simulink model "Dpt_S_Fun_1_C"  (Simulink 4.00)
settings: Solver=ode45  SolverMode=SingleTasking  StartTime=0.0  StopTime=0.4  FixedStep=0.01  MaxStep=0.001  RelTol=1e-3  AbsTol=1e-3
PreLoadFcn:
  | Load_Param_1
undefined symbols (not defined in the file): Cm, Cw, Fi, J, L, Mnabr, R, Tnabr, V
settings Model: SaveTime=off  SaveOutput=off  LimitDataPoints=off  RTWTemplateMakefile=grt_vc.tmf  BlockReductionOpt=off

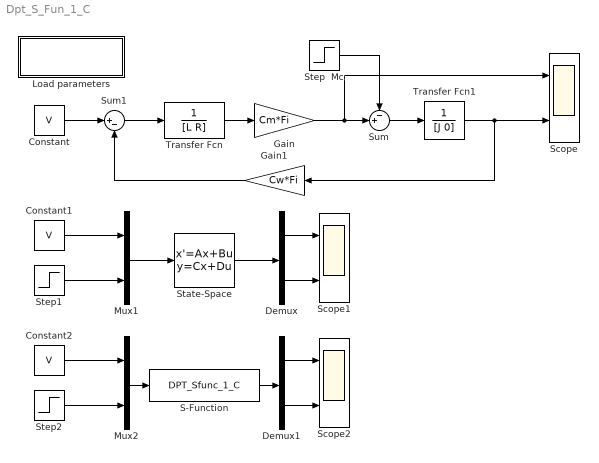
== system Dpt_S_Fun_1_C ==
  Constant : Constant  Value=V
  Constant1 : Constant  Value=V
  Constant2 : Constant  Value=V
  Demux : Demux  Outputs=2  BusSelectionMode=off
  Demux1 : Demux  Outputs=2  BusSelectionMode=off
  Gain : Gain  Gain=Cm*Fi  Multiplication=Element-wise(K.*u)  SaturateOnIntegerOverflow=on
  Gain1 : Gain  Orientation=left  Gain=Cw*Fi  Multiplication=Element-wise(K.*u)  SaturateOnIntegerOverflow=on
  Load parameters : Subsystem
      settings: OpenFcn=Load_Param_1  RTWFcnNameOpts=Auto  RTWFileNameOpts=Auto
      mask Help: Click here to save t and yout in an ascii data file called temp.dat
      mask Display: disp('Click here to\n load parameters')
  Mux1 : Mux  Inputs=2
  Mux2 : Mux  Inputs=2
  S-Function : S-Function  FunctionName=DPT_Sfunc_1_C  Parameters=L,R,J,Cm,Cw,Fi  PortCounts=[]  SFunctionModules=''
  Scope : Scope  NumInputPorts=2
      settings: TimeRange=0.4  YMin=-3286.73~0  YMax=12937.8~30  SaveToWorkspace=off  SaveName=ScopeData  LimitDataPoints=on  MaxDataPoints=5000
  Scope1 : Scope  NumInputPorts=2
      settings: TimeRange=0.4  YMin=-3286.73~0  YMax=12937.8~30  SaveToWorkspace=off  LimitDataPoints=on  MaxDataPoints=5000
  Scope2 : Scope  NumInputPorts=2
      settings: TimeRange=0.4  YMin=-3286.73~0  YMax=12937.8~30  SaveToWorkspace=off  SaveName=ScopeData2  LimitDataPoints=on  MaxDataPoints=5000
  State-Space : StateSpace  A=[-R/L -Cw*Fi/L;Cm*Fi/J 0]  B=[1/L 0;0 -1/J]  C=[Cm*Fi 0;0 1]  D=[0 0;0 0]  X0=[0;0]  AbsoluteTolerance=auto  Realization=auto
  Step  Mc : Step  Time=Tnabr  Before=0  After=Mnabr  SampleTime=0
  Step1 : Step  Time=Tnabr  Before=0  After=Mnabr  SampleTime=0
  Step2 : Step  Time=Tnabr  Before=0  After=Mnabr  SampleTime=0
  Sum : Sum  Inputs=-+|  SaturateOnIntegerOverflow=on
  Sum1 : Sum  Inputs=|+-  SaturateOnIntegerOverflow=on
  Transfer Fcn : TransferFcn  Numerator=[1]  Denominator=[L R]  AbsoluteTolerance=auto  Realization=auto
  Transfer Fcn1 : TransferFcn  Numerator=[1]  Denominator=[J 0]  AbsoluteTolerance=auto  Realization=auto
  wires:
  Constant2/1 -> Mux2/1
  Step2/1 -> Mux2/2
  Mux2/1 -> S-Function/1
  Demux1/1 -> Scope2/1
  Demux1/2 -> Scope2/2
  S-Function/1 -> Demux1/1
  Constant/1 -> Sum1/1
  Sum1/1 -> Transfer Fcn/1
  Step  Mc/1 -> Sum/1
  Sum/1 -> Transfer Fcn1/1
  Transfer Fcn/1 -> Gain/1
  Gain/1 -> Sum/2, Scope/1
  Transfer Fcn1/1 -> Gain1/1, Scope/2
  Gain1/1 -> Sum1/2
  Demux/1 -> Scope1/1
  Demux/2 -> Scope1/2
  State-Space/1 -> Demux/1
  Constant1/1 -> Mux1/1
  Step1/1 -> Mux1/2
  Mux1/1 -> State-Space/1

== system Dpt_S_Fun_1_C/Load parameters ==
  note: a
